simulink model "speed_pi_model"  (R2023b)
settings: Solver=FixedStepDiscrete  StartTime=0.0  StopTime=0.001  FixedStep=0.0001  RelTol=1e-3
values from neighbouring files (symbols this model uses):
  Kaw_speed = 125.66370391845703    [speed_pi_interface.sldd]
  Ki_speed = 22.110023498535156    [speed_pi_interface.sldd]
  Kp_speed = 0.34031936526298523    [speed_pi_interface.sldd]
settings Model: DataDictionary=speed_pi_interface.sldd  Creator=user  LastModifiedBy=user
settings OptimizationCC: EnhancedBackFolding=on  PassReuseOutputArgsAs=Individual arguments  OptimizeBlockOrder=speed  DifferentSizesBufferReuse=on  OptimizationCustomize=off  EfficientTunableParamExpr=on
settings DebuggingCC: ParameterPrecisionLossMsg=none  ParameterTunabilityLossMsg=error
settings HardwareCC: ProdBitPerPointer=32  ProdBitPerSizeT=32  ProdBitPerPtrDiffT=32  ProdLargestAtomicInteger=Long  ProdLargestAtomicFloat=Double  ProdWordSize=32  ProdHWDeviceType=ARM Compatible->ARM Cortex  TargetLargestAtomicInteger=Long  TargetLargestAtomicFloat=Double  TargetIntDivRoundTo=Zero  TargetEndianess=LittleEndian  TargetHWDeviceType=ARM Compatible->ARM Cortex  ProdEqTarget=off
settings SFSimCC: MATLABDynamicMemAlloc=off
settings RTWCC: Description=Embedded Coder  SystemTargetFile=ert.tlc  GenCodeOnly=on  TemplateMakefile=ert_default_tmf  GenerateReport=on
settings CodeAppCC: ForceParamTrailComments=on  IgnoreCustomStorageClasses=off  OperatorAnnotations=on  SimulinkDataObjDesc=on  SFDataObjDesc=on  InsertBlockDesc=on
settings ERTTargetCC: TargetLangStandard=C99 (ISO)  CodeInterfacePackaging=Reusable function  ERTCustomFileTemplate=example_file_process.tlc

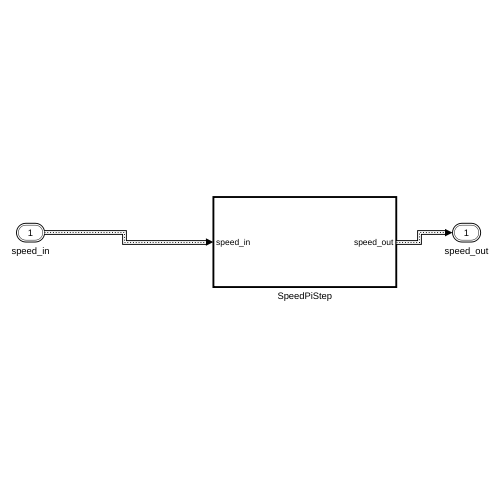
[thumbnail: Simulink's stored preview of the top-level diagram]
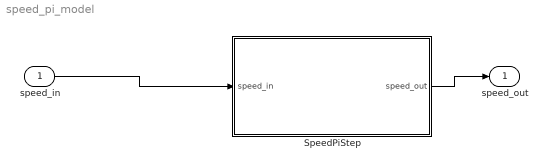
== system speed_pi_model ==
  speed_in : Inport  OutDataTypeStr=Bus: speed_pi_input_t  BusOutputAsStruct=on
  SpeedPiStep : Subsystem  TreatAsAtomicUnit=on  RTWFcnName=SpeedPiStep  RTWFileName=SpeedPiStep
      settings: RTWFcnNameOpts=User specified  RTWFileNameOpts=User specified
  speed_out : Outport  OutDataTypeStr=Bus: speed_pi_output_t
  wires:
  speed_in/1 -> SpeedPiStep/1(speed_in)
  SpeedPiStep/1(speed_out) -> speed_out/1

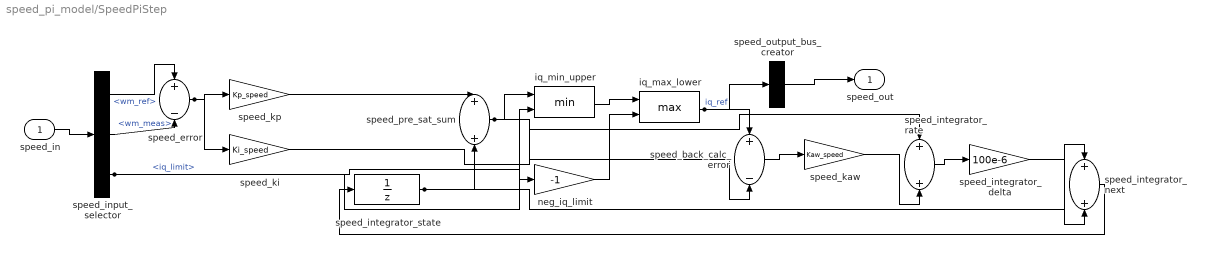
== system speed_pi_model/SpeedPiStep ==
  speed_in : Inport  OutDataTypeStr=Bus: speed_pi_input_t  BusOutputAsStruct=on
  iq_max_lower : MinMax  Function=max  Inputs=2
  iq_min_upper : MinMax  Inputs=2
  neg_iq_limit : Gain  Gain=-1  ParamDataTypeStr=T_SpeedPiFloat  OutDataTypeStr=T_SpeedPiCurrent
  speed_back_calc_error : Sum  Inputs=+-  OutDataTypeStr=T_SpeedPiCurrent  AccumDataTypeStr=T_SpeedPiCurrent
  speed_error : Sum  Inputs=+-  OutDataTypeStr=T_SpeedPiSpeed  AccumDataTypeStr=T_SpeedPiSpeed
  speed_input_selector : BusSelector  OutputSignals=wm_ref,wm_meas,iq_limit
  speed_integrator_delta : Gain  Gain=100e-6  ParamDataTypeStr=T_SpeedPiFloat  OutDataTypeStr=T_SpeedPiCurrent
  speed_integrator_next : Sum  OutDataTypeStr=T_SpeedPiCurrent  AccumDataTypeStr=T_SpeedPiCurrent
  speed_integrator_rate : Sum  OutDataTypeStr=T_SpeedPiCurrent  AccumDataTypeStr=T_SpeedPiCurrent
  speed_integrator_state : UnitDelay  SampleTime=100e-6  HasFrameUpgradeWarning=on
  speed_kaw : Gain  Gain=Kaw_speed  ParamDataTypeStr=T_SpeedPiGain  OutDataTypeStr=T_SpeedPiCurrent
  speed_ki : Gain  Gain=Ki_speed  ParamDataTypeStr=T_SpeedPiGain  OutDataTypeStr=T_SpeedPiCurrent
  speed_kp : Gain  Gain=Kp_speed  ParamDataTypeStr=T_SpeedPiGain  OutDataTypeStr=T_SpeedPiCurrent
  speed_output_bus_creator : BusCreator  Inputs=1  OutDataTypeStr=Bus: speed_pi_output_t  NonVirtualBus=on
  speed_pre_sat_sum : Sum  OutDataTypeStr=T_SpeedPiCurrent  AccumDataTypeStr=T_SpeedPiCurrent
  speed_out : Outport  OutDataTypeStr=Bus: speed_pi_output_t
  wires:
  speed_in/1 -> speed_input_selector/1
  speed_input_selector/1 -> speed_error/1  "<wm_ref>"
  speed_input_selector/2 -> speed_error/2  "<wm_meas>"
  speed_error/1 -> speed_kp/1, speed_ki/1
  speed_kp/1 -> speed_pre_sat_sum/1
  speed_integrator_state/1 -> speed_pre_sat_sum/2, speed_integrator_next/1
  speed_pre_sat_sum/1 -> iq_min_upper/1, speed_back_calc_error/2
  speed_input_selector/3 -> iq_min_upper/2, neg_iq_limit/1  "<iq_limit>"
  iq_min_upper/1 -> iq_max_lower/1
  neg_iq_limit/1 -> iq_max_lower/2
  iq_max_lower/1 -> speed_output_bus_creator/1, speed_back_calc_error/1  "iq_ref"
  speed_output_bus_creator/1 -> speed_out/1
  speed_back_calc_error/1 -> speed_kaw/1
  speed_ki/1 -> speed_integrator_rate/1
  speed_kaw/1 -> speed_integrator_rate/2
  speed_integrator_rate/1 -> speed_integrator_delta/1
  speed_integrator_delta/1 -> speed_integrator_next/2
  speed_integrator_next/1 -> speed_integrator_state/1
